simulink model "WristIdentScheme"  (R2025b)
settings: Solver=FixedStepAuto  StartTime=0.0  StopTime=10  FixedStep=1e-3  RelTol=1e-3
model workspace: external: MATLAB File WristAssembly_DataFile.m (data not in the file)
undefined symbols (not defined in the file): smiData, X, Y, Z
libraries: sm_lib x20, nesl_utility x16
settings Model: Creator=Asus  LastModifiedBy=Asus

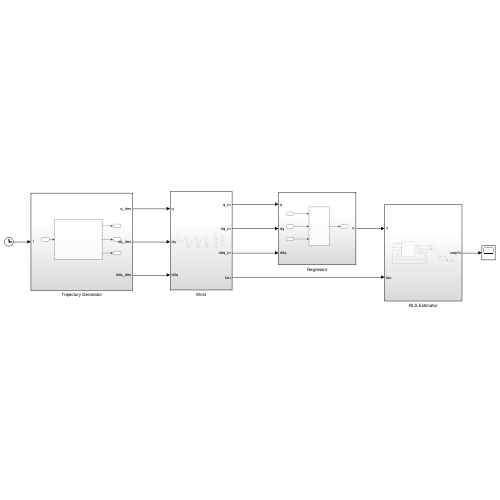
[thumbnail: Simulink's stored preview of the top-level diagram]
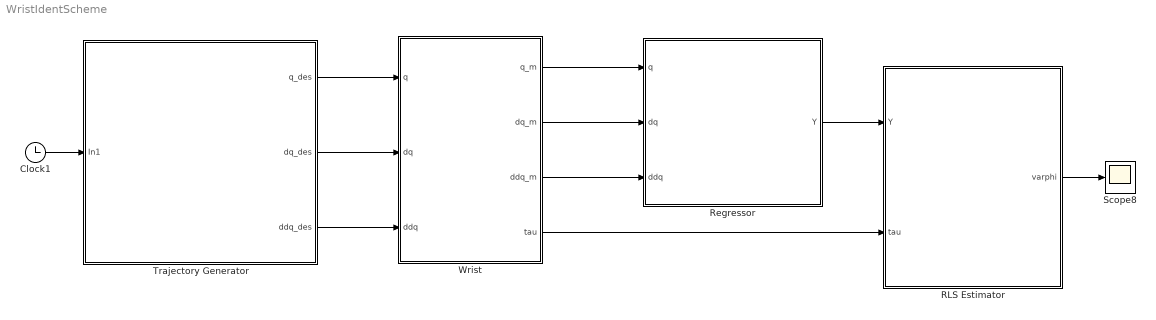
== system WristIdentScheme ==
  Clock1 : Clock
  RLS Estimator : Subsystem
  Regressor : Subsystem
  Scope8 : Scope
      settings: ActiveDisplayYMinimum=-8.9167917961157173  ActiveDisplayYMaximum=6.4052375907209349  DataLoggingVariableName=ScopeData12
  Trajectory Generator : Subsystem
  Wrist : Subsystem
  wires:
  Regressor/1(Y) -> RLS Estimator/1(Y)
  RLS Estimator/1(varphi) -> Scope8/1
  Wrist/1(q_m) -> Regressor/1(q)
  Wrist/2(dq_m) -> Regressor/2(dq)
  Wrist/3(ddq_m) -> Regressor/3(ddq)
  Wrist/4(tau) -> RLS Estimator/2(tau)
  Clock1/1 -> Trajectory Generator/1(In1)
  Trajectory Generator/2(dq_des) -> Wrist/2(dq)
  Trajectory Generator/1(q_des) -> Wrist/1(q)
  Trajectory Generator/3(ddq_des) -> Wrist/3(ddq)

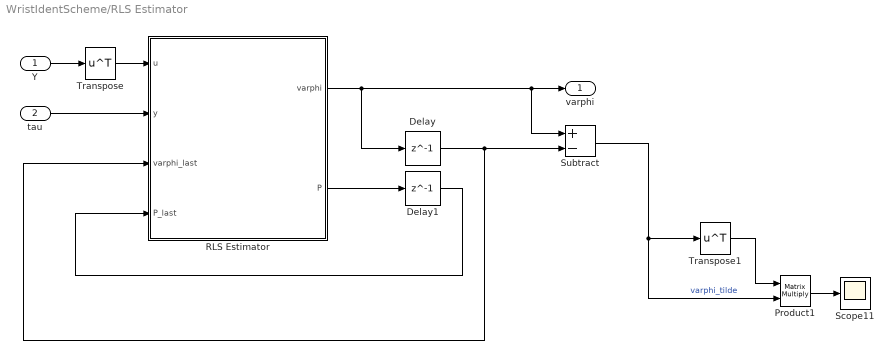
== system WristIdentScheme/RLS Estimator ==
  Y : Inport
  tau : Inport  Port=2
  Delay : Delay  DelayLength=1  InitialCondition=zeros(12, 1)
  Delay1 : Delay  DelayLength=1  InitialCondition=1e+4 * eye(12)
  Product1 : Product  Multiplication=Matrix(*)
  RLS Estimator : MATLAB Function  TreatAsAtomicUnit=on
  Scope11 : Scope
      settings: ActiveDisplayYMinimum=-1.1979056789064427E-9  ActiveDisplayYMaximum=5.9268912686595225E-10  DataLoggingVariableName=ScopeData14
  Subtract : Sum  Inputs=+-
  Transpose : Math  Operator=transpose
  Transpose1 : Math  Operator=transpose
  varphi : Outport
  wires:
  Y/1 -> Transpose/1
  tau/1 -> RLS Estimator/2(y)
  RLS Estimator/1(varphi) -> Subtract/1, varphi/1, Delay/1
  Delay/1 -> RLS Estimator/3(varphi_last), Subtract/2
  RLS Estimator/2(P) -> Delay1/1
  Delay1/1 -> RLS Estimator/4(P_last)
  Transpose/1 -> RLS Estimator/1(u)
  Transpose1/1 -> Product1/1
  Product1/1 -> Scope11/1
  Subtract/1 -> Transpose1/1, Product1/2  "varphi_tilde"

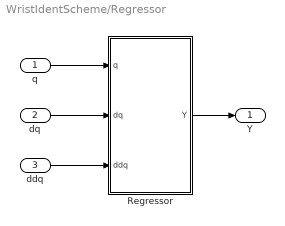
== system WristIdentScheme/Regressor ==
  q : Inport
  dq : Inport  Port=2
  ddq : Inport  Port=3
  Regressor : MATLAB Function  TreatAsAtomicUnit=on
  Y : Outport
  wires:
  q/1 -> Regressor/1(q)
  dq/1 -> Regressor/2(dq)
  ddq/1 -> Regressor/3(ddq)
  Regressor/1(Y) -> Y/1

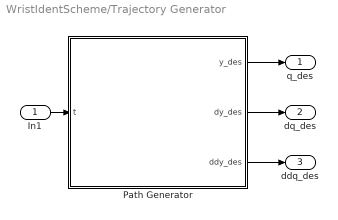
== system WristIdentScheme/Trajectory Generator ==
  In1 : Inport
  Path Generator : MATLAB Function  TreatAsAtomicUnit=on
  q_des : Outport
  dq_des : Outport  Port=2
  ddq_des : Outport  Port=3
  wires:
  In1/1 -> Path Generator/1(t)
  Path Generator/1(y_des) -> q_des/1
  Path Generator/2(dy_des) -> dq_des/1
  Path Generator/3(ddy_des) -> ddq_des/1

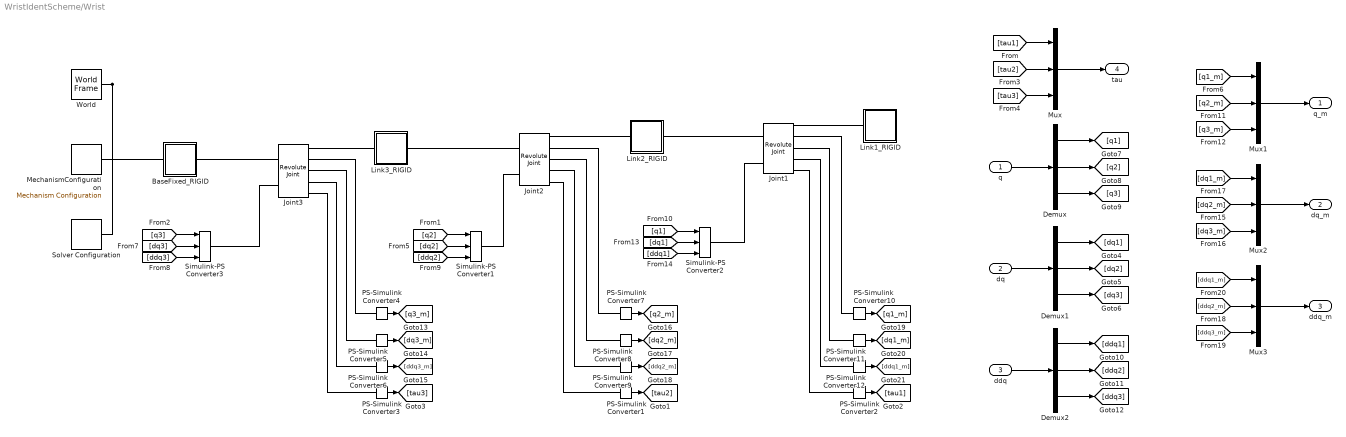
== system WristIdentScheme/Wrist ==
  q : Inport
  dq : Inport  Port=2
  ddq : Inport  Port=3
  BaseFixed_RIGID : Subsystem
  Demux : Demux  Outputs=3
  Demux1 : Demux  Outputs=3
  Demux2 : Demux  Outputs=3
  Joint1 : sm_lib/Joints/Revolute Joint  JointMode=Normal  CompositeWrenchDir=FollowerOnBase  CompositeWrenchFrame=BaseFrame  SenseConstraintForce=off  SenseConstraintTorque=off  SenseTotalForce=off  SenseTotalTorque=off  PositionTargetSpecify=on  PositionTargetPriority=Low  PositionTargetValue=smiData.RevoluteJoint(1).Rz.Pos  PositionTargetValueUnits=deg  VelocityTargetSpecify=off  VelocityTargetPriority=High  VelocityTargetValue=0  VelocityTargetValueUnits=deg/s  EquilibriumPosition=0  EquilibriumPositionUnits=deg  SpringStiffness=0  SpringStiffnessUnits=N*m/deg  DampingCoefficient=0  DampingCoefficientUnits=N*m/(deg/s)  LowerLimitSpecify=off  LowerLimitBound=-90  LowerLimitBoundUnits=deg  LowerLimitStiffness=1e4  LowerLimitStiffnessUnits=N*m/deg  LowerLimitDamping=10  LowerLimitDampingUnits=N*m/(deg/s)  LowerLimitTransitionRegionWidth=0.1  LowerLimitTransitionRegionWidthUnits=deg  UpperLimitSpecify=off  UpperLimitBound=90  UpperLimitBoundUnits=deg  UpperLimitStiffness=1e4  UpperLimitStiffnessUnits=N*m/deg  UpperLimitDamping=10  UpperLimitDampingUnits=N*m/(deg/s)  UpperLimitTransitionRegionWidth=0.1  UpperLimitTransitionRegionWidthUnits=deg  TorqueActuationMode=ComputedTorque  MotionActuationMode=InputMotion  SensePosition=on  SenseVelocity=on  SenseAcceleration=on  SenseTorqueForce=on  SenseLowerLimitTorqueForce=off  SenseUpperLimitTorqueForce=off
  Joint2 : sm_lib/Joints/Revolute Joint  JointMode=Normal  CompositeWrenchDir=FollowerOnBase  CompositeWrenchFrame=BaseFrame  SenseConstraintForce=off  SenseConstraintTorque=off  SenseTotalForce=off  SenseTotalTorque=off  PositionTargetSpecify=on  PositionTargetPriority=Low  PositionTargetValue=smiData.RevoluteJoint(2).Rz.Pos  PositionTargetValueUnits=deg  VelocityTargetSpecify=off  VelocityTargetPriority=High  VelocityTargetValue=0  VelocityTargetValueUnits=deg/s  EquilibriumPosition=0  EquilibriumPositionUnits=deg  SpringStiffness=0  SpringStiffnessUnits=N*m/deg  DampingCoefficient=0  DampingCoefficientUnits=N*m/(deg/s)  LowerLimitSpecify=off  LowerLimitBound=-90  LowerLimitBoundUnits=deg  LowerLimitStiffness=1e4  LowerLimitStiffnessUnits=N*m/deg  LowerLimitDamping=10  LowerLimitDampingUnits=N*m/(deg/s)  LowerLimitTransitionRegionWidth=0.1  LowerLimitTransitionRegionWidthUnits=deg  UpperLimitSpecify=off  UpperLimitBound=90  UpperLimitBoundUnits=deg  UpperLimitStiffness=1e4  UpperLimitStiffnessUnits=N*m/deg  UpperLimitDamping=10  UpperLimitDampingUnits=N*m/(deg/s)  UpperLimitTransitionRegionWidth=0.1  UpperLimitTransitionRegionWidthUnits=deg  TorqueActuationMode=ComputedTorque  MotionActuationMode=InputMotion  SensePosition=on  SenseVelocity=on  SenseAcceleration=on  SenseTorqueForce=on  SenseLowerLimitTorqueForce=off  SenseUpperLimitTorqueForce=off
  Joint3 : sm_lib/Joints/Revolute Joint  JointMode=Normal  CompositeWrenchDir=FollowerOnBase  CompositeWrenchFrame=BaseFrame  SenseConstraintForce=off  SenseConstraintTorque=off  SenseTotalForce=off  SenseTotalTorque=off  PositionTargetSpecify=on  PositionTargetPriority=Low  PositionTargetValue=smiData.RevoluteJoint(3).Rz.Pos  PositionTargetValueUnits=deg  VelocityTargetSpecify=off  VelocityTargetPriority=High  VelocityTargetValue=0  VelocityTargetValueUnits=deg/s  EquilibriumPosition=0  EquilibriumPositionUnits=deg  SpringStiffness=0  SpringStiffnessUnits=N*m/deg  DampingCoefficient=0  DampingCoefficientUnits=N*m/(deg/s)  LowerLimitSpecify=off  LowerLimitBound=-90  LowerLimitBoundUnits=deg  LowerLimitStiffness=1e4  LowerLimitStiffnessUnits=N*m/deg  LowerLimitDamping=10  LowerLimitDampingUnits=N*m/(deg/s)  LowerLimitTransitionRegionWidth=0.1  LowerLimitTransitionRegionWidthUnits=deg  UpperLimitSpecify=off  UpperLimitBound=90  UpperLimitBoundUnits=deg  UpperLimitStiffness=1e4  UpperLimitStiffnessUnits=N*m/deg  UpperLimitDamping=10  UpperLimitDampingUnits=N*m/(deg/s)  UpperLimitTransitionRegionWidth=0.1  UpperLimitTransitionRegionWidthUnits=deg  TorqueActuationMode=ComputedTorque  MotionActuationMode=InputMotion  SensePosition=on  SenseVelocity=on  SenseAcceleration=on  SenseTorqueForce=on  SenseLowerLimitTorqueForce=off  SenseUpperLimitTorqueForce=off
  Link1_RIGID : Subsystem
  Link2_RIGID : Subsystem
  Link3_RIGID : Subsystem
  MechanismConfiguration : sm_lib/Utilities/Mechanism Configuration  UniformGravity=Constant  GravityVector=[0 0 -9.80665] * 1  GravityVectorUnits=m/s^2  LinearizationDelta=0.001  JointModeTransitionNonlinearIterations=2
  Mux{,1..3} (4 alike) : Mux  Inputs=3
  PS-Simulink Converter1 : nesl_utility/PS-Simulink Converter  PhysicalDomain=network_engine_domain  SubClassName=ps_output  LeftPortType=input  RightPortType=output  PseudoPeriodic=off  Frequencies=[]  VectorFormat=inherit  Unit=N*m  AffineConversion=off
  PS-Simulink Converter10 : nesl_utility/PS-Simulink Converter  PhysicalDomain=network_engine_domain  SubClassName=ps_output  LeftPortType=input  RightPortType=output  PseudoPeriodic=off  Frequencies=[]  VectorFormat=inherit  Unit=rad  AffineConversion=off
  PS-Simulink Converter11 : nesl_utility/PS-Simulink Converter  PhysicalDomain=network_engine_domain  SubClassName=ps_output  LeftPortType=input  RightPortType=output  PseudoPeriodic=off  Frequencies=[]  VectorFormat=inherit  Unit=rad/s  AffineConversion=off
  PS-Simulink Converter12 : nesl_utility/PS-Simulink Converter  PhysicalDomain=network_engine_domain  SubClassName=ps_output  LeftPortType=input  RightPortType=output  PseudoPeriodic=off  Frequencies=[]  VectorFormat=inherit  Unit=rad/s^2  AffineConversion=off
  PS-Simulink Converter2 : nesl_utility/PS-Simulink Converter  PhysicalDomain=network_engine_domain  SubClassName=ps_output  LeftPortType=input  RightPortType=output  PseudoPeriodic=off  Frequencies=[]  VectorFormat=inherit  Unit=N*m  AffineConversion=off
  PS-Simulink Converter3 : nesl_utility/PS-Simulink Converter  PhysicalDomain=network_engine_domain  SubClassName=ps_output  LeftPortType=input  RightPortType=output  PseudoPeriodic=off  Frequencies=[]  VectorFormat=inherit  Unit=N*m  AffineConversion=off
  PS-Simulink Converter4 : nesl_utility/PS-Simulink Converter  PhysicalDomain=network_engine_domain  SubClassName=ps_output  LeftPortType=input  RightPortType=output  PseudoPeriodic=off  Frequencies=[]  VectorFormat=inherit  Unit=rad  AffineConversion=off
  PS-Simulink Converter5 : nesl_utility/PS-Simulink Converter  PhysicalDomain=network_engine_domain  SubClassName=ps_output  LeftPortType=input  RightPortType=output  PseudoPeriodic=off  Frequencies=[]  VectorFormat=inherit  Unit=rad/s  AffineConversion=off
  PS-Simulink Converter6 : nesl_utility/PS-Simulink Converter  PhysicalDomain=network_engine_domain  SubClassName=ps_output  LeftPortType=input  RightPortType=output  PseudoPeriodic=off  Frequencies=[]  VectorFormat=inherit  Unit=rad/s^2  AffineConversion=off
  PS-Simulink Converter7 : nesl_utility/PS-Simulink Converter  PhysicalDomain=network_engine_domain  SubClassName=ps_output  LeftPortType=input  RightPortType=output  PseudoPeriodic=off  Frequencies=[]  VectorFormat=inherit  Unit=rad  AffineConversion=off
  PS-Simulink Converter8 : nesl_utility/PS-Simulink Converter  PhysicalDomain=network_engine_domain  SubClassName=ps_output  LeftPortType=input  RightPortType=output  PseudoPeriodic=off  Frequencies=[]  VectorFormat=inherit  Unit=rad/s  AffineConversion=off
  PS-Simulink Converter9 : nesl_utility/PS-Simulink Converter  PhysicalDomain=network_engine_domain  SubClassName=ps_output  LeftPortType=input  RightPortType=output  PseudoPeriodic=off  Frequencies=[]  VectorFormat=inherit  Unit=rad/s^2  AffineConversion=off
  Simulink-PS Converter1 : nesl_utility/Simulink-PS Converter  PhysicalDomain=network_engine_domain  SubClassName=ps_input  LeftPortType=input  RightPortType=output  PseudoPeriodic=off  Frequencies=[]  NoiseDistribution=none  NoiseParameters=[]  Unit=rad  AffineConversion=off  FilteringAndDerivatives=provide  SimscapeFilterOrder=1  InputFilterTimeConstant=0.001  UdotUserProvided=2
  Simulink-PS Converter2 : nesl_utility/Simulink-PS Converter  PhysicalDomain=network_engine_domain  SubClassName=ps_input  LeftPortType=input  RightPortType=output  PseudoPeriodic=off  Frequencies=[]  NoiseDistribution=none  NoiseParameters=[]  Unit=rad  AffineConversion=off  FilteringAndDerivatives=provide  SimscapeFilterOrder=1  InputFilterTimeConstant=0.001  UdotUserProvided=2
  Simulink-PS Converter3 : nesl_utility/Simulink-PS Converter  PhysicalDomain=network_engine_domain  SubClassName=ps_input  LeftPortType=input  RightPortType=output  PseudoPeriodic=off  Frequencies=[]  NoiseDistribution=none  NoiseParameters=[]  Unit=rad  AffineConversion=off  FilteringAndDerivatives=provide  SimscapeFilterOrder=1  InputFilterTimeConstant=0.001  UdotUserProvided=2
  Solver Configuration : nesl_utility/Solver Configuration  PhysicalDomain=network_engine_domain  SubClassName=solver  LeftPortType=input  RightPortType=generic  Tones=[]  Harmonics=[]  SimulateNoise=off  Profile=off  UseLocalSampling=off  EnableSwitchedLinearOptims=on  FrequencyDomain=off  UseCCode=off  RelTol=0.001  AbsTol=0.001  MinStep=1e-09  ToWorkspace=off  RevertToSquareIcSolve=off  NumHomotopyIterations=100  PhasorMode=off  PhasorModeNumHarmonics=1  ConsistencySolver=NEWTON_XTOL_AFTER_FTOL  IndexReductionMethod=DerivativeReplacement  DoDC=off  ResidualTolerance=1e-09  ConsistencyTolSource=GLOBAL  ConsistencyAbsTol=0.001  ConsistencyRelTol=0.001  ConsistencyTolFactor=0.001  UseLocalSolver=off  LocalSolverChoice=NE_BACKWARD_EULER_ADVANCER  ResolveIndetEquations=on  FunctionEvalNumThread=1  LocalSolverSampleTime=0.001  DoFixedCost=off  MaxNonlinIter=3  MaxModeIter=2  ComputeImpulses=off  ImpulseIterations=2  LinearAlgebra=auto  LinearAlgebraNumThread=0  EquationFormulation=NE_TIME_EF  DelaysMemoryBudget=1024  AutomaticFiltering=on  FilteringTimeConstant=0.001  PartitionStorageMethod=AS_NEEDED  PartitionMemoryBudget=1024  PartitionMethod=ROBUST  MultibodyUseLocalSolver=off  MultibodyLocalSolverChoice=ODE1  MultibodyLocalSolverSampleTime=0.001
  World : sm_lib/Frames and Transforms/World Frame
  q_m : Outport
  dq_m : Outport  Port=2
  ddq_m : Outport  Port=3
  tau : Outport  Port=4
  wires:
  PS-Simulink Converter3/1 -> [tau3]
  PS-Simulink Converter1/1 -> [tau2]
  PS-Simulink Converter2/1 -> [tau1]
  [tau3] -> Mux/3
  Mux/1 -> tau/1
  Demux2/3 -> [ddq3]
  Demux1/2 -> [dq2]
  Demux/3 -> [q3]
  q/1 -> Demux/1
  ddq/1 -> Demux2/1
  Demux/2 -> [q2]
  Demux1/1 -> [dq1]
  [tau2] -> Mux/2
  Demux/1 -> [q1]
  Demux2/1 -> [ddq1]
  Demux2/2 -> [ddq2]
  Demux1/3 -> [dq3]
  [tau1] -> Mux/1
  dq/1 -> Demux1/1
  PS-Simulink Converter4/1 -> [q3_m]
  PS-Simulink Converter5/1 -> [dq3_m]
  PS-Simulink Converter6/1 -> [ddq3_m]
  PS-Simulink Converter9/1 -> [ddq2_m]
  PS-Simulink Converter7/1 -> [q2_m]
  PS-Simulink Converter8/1 -> [dq2_m]
  PS-Simulink Converter12/1 -> [ddq1_m]
  PS-Simulink Converter10/1 -> [q1_m]
  PS-Simulink Converter11/1 -> [dq1_m]
  Mux1/1 -> q_m/1
  [q1_m] -> Mux1/1
  [q2_m] -> Mux1/2
  [q3_m] -> Mux1/3
  Mux2/1 -> dq_m/1
  [dq1_m] -> Mux2/1
  [dq3_m] -> Mux2/3
  [dq2_m] -> Mux2/2
  [ddq1_m] -> Mux3/1
  Mux3/1 -> ddq_m/1
  [ddq3_m] -> Mux3/3
  [ddq2_m] -> Mux3/2
  [q3] -> Simulink-PS Converter3/1
  [dq3] -> Simulink-PS Converter3/2
  [ddq3] -> Simulink-PS Converter3/3
  [dq2] -> Simulink-PS Converter1/2
  [q2] -> Simulink-PS Converter1/1
  [ddq2] -> Simulink-PS Converter1/3
  [q1] -> Simulink-PS Converter2/1
  [ddq1] -> Simulink-PS Converter2/3
  [dq1] -> Simulink-PS Converter2/2
  connections:
  Link3_RIGID/RConn1 -- Joint2/LConn1
  World/RConn1 -- BaseFixed_RIGID/LConn1 -- Solver Configuration/RConn1 -- MechanismConfiguration/RConn1
  BaseFixed_RIGID/RConn1 -- Joint3/LConn1
  Link2_RIGID/RConn1 -- Joint1/LConn1
  Link3_RIGID/LConn1 -- Joint3/RConn1
  Link2_RIGID/LConn1 -- Joint2/RConn1
  Link1_RIGID/LConn1 -- Joint1/RConn1
  Simulink-PS Converter3/RConn1 -- Joint3/LConn2
  PS-Simulink Converter3/LConn1 -- Joint3/RConn5
  Simulink-PS Converter1/RConn1 -- Joint2/LConn2
  PS-Simulink Converter1/LConn1 -- Joint2/RConn5
  Simulink-PS Converter2/RConn1 -- Joint1/LConn2
  PS-Simulink Converter2/LConn1 -- Joint1/RConn5
  PS-Simulink Converter4/LConn1 -- Joint3/RConn2
  PS-Simulink Converter5/LConn1 -- Joint3/RConn3
  PS-Simulink Converter6/LConn1 -- Joint3/RConn4
  PS-Simulink Converter7/LConn1 -- Joint2/RConn2
  PS-Simulink Converter8/LConn1 -- Joint2/RConn3
  PS-Simulink Converter9/LConn1 -- Joint2/RConn4
  PS-Simulink Converter10/LConn1 -- Joint1/RConn2
  PS-Simulink Converter11/LConn1 -- Joint1/RConn3
  PS-Simulink Converter12/LConn1 -- Joint1/RConn4

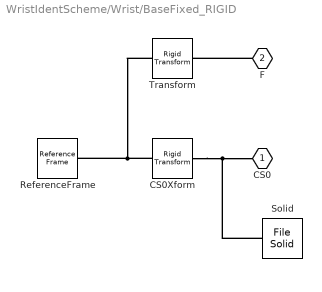
== system WristIdentScheme/Wrist/BaseFixed_RIGID ==
  CS0Xform : sm_lib/Frames and Transforms/Rigid Transform  RotationMethod=ArbitraryAxis  FollAlignAxisA=+X  BaseAlignAxisA=+Y  FollAlignAxisB=+Y  BaseAlignAxisB=+Z  RotationStandardAxis=+Z  RotationAngle=smiData.RigidTransform(3).angle  RotationAngleUnits=rad  RotationArbitraryAxis=smiData.RigidTransform(3).axis  RotationSequenceAxes=FollowerAxes  RotationSequence=XYX  RotationSequenceAngles=[0 0 0]  RotationSequenceAnglesUnits=deg  RotationMatrix=[1 0 0;0 1 0;0 0 1]  Quaternion=[1 0 0 0]  TranslationMethod=Cartesian  TranslationCartesianOffset=smiData.RigidTransform(3).translation  TranslationCartesianOffsetUnits=mm  TranslationStandardAxis=+Z  TranslationStandardOffset=0  TranslationStandardOffsetUnits=m  TranslationROffset=0  TranslationROffsetUnits=m  TranslationThetaOffset=0  TranslationThetaOffsetUnits=deg  TranslationZOffset=0  TranslationZOffsetUnits=m
  ReferenceFrame : sm_lib/Frames and Transforms/Reference Frame
  Solid : sm_lib/Body Elements/File Solid  ExtGeomFileName=BaseFixed.STEP  UnitType=FromFile  ExtGeomFileUnits=m  StepReaderType=HEX  ExportConvexHullGeometry=off  InertiaType=Custom  BasedOnType=DensityFromFile  Density=1000  DensityUnits=kg/m^3  Mass=smiData.BaseFixed.mass  MassUnits=kg  CenterOfMass=smiData.BaseFixed.CoM  CenterOfMassUnits=mm  MomentsOfInertia=smiData.BaseFixed.MoI  MomentsOfInertiaUnits=kg*mm^2  ProductsOfInertia=smiData.BaseFixed.PoI  ProductsOfInertiaUnits=kg*mm^2  GraphicType=FromGeometry  MarkerShape=Sphere  MarkerSize=10  GraphicVisPropType=SimpleVisualProperties  GraphicDiffuseColor=smiData.Solid(14).color  GraphicOpacity=smiData.Solid(14).opacity  GraphicSpecularColor=[0.5 0.5 0.5 1.0]  GraphicAmbientColor=[0.15 0.15 0.15 1.0]  GraphicEmissiveColor=[0.0 0.0 0.0 1.0]  GraphicShininess=75  DoExposeReferenceFrame=on  SerializedFrames=<Frames/>
  Transform : sm_lib/Frames and Transforms/Rigid Transform  RotationMethod=ArbitraryAxis  FollAlignAxisA=+X  BaseAlignAxisA=+Y  FollAlignAxisB=+Y  BaseAlignAxisB=+Z  RotationStandardAxis=+Z  RotationAngle=smiData.RigidTransform(10).angle  RotationAngleUnits=rad  RotationArbitraryAxis=smiData.RigidTransform(10).axis  RotationSequenceAxes=FollowerAxes  RotationSequence=XYX  RotationSequenceAngles=[0 0 0]  RotationSequenceAnglesUnits=deg  RotationMatrix=[1 0 0;0 1 0;0 0 1]  Quaternion=[1 0 0 0]  TranslationMethod=Cartesian  TranslationCartesianOffset=smiData.RigidTransform(10).translation  TranslationCartesianOffsetUnits=mm  TranslationStandardAxis=+Z  TranslationStandardOffset=0  TranslationStandardOffsetUnits=m  TranslationROffset=0  TranslationROffsetUnits=m  TranslationThetaOffset=0  TranslationThetaOffsetUnits=deg  TranslationZOffset=0  TranslationZOffsetUnits=m
  CS0 : PMIOPort  Side=Left
  F : PMIOPort  Port=2  Side=Right
  connections:
  CS0Xform/RConn1 -- Solid/RConn1 -- CS0/RConn1
  CS0Xform/LConn1 -- Transform/LConn1 -- ReferenceFrame/RConn1
  F/RConn1 -- Transform/RConn1

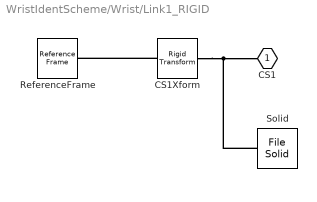
== system WristIdentScheme/Wrist/Link1_RIGID ==
  CS1Xform : sm_lib/Frames and Transforms/Rigid Transform  RotationMethod=ArbitraryAxis  FollAlignAxisA=+X  BaseAlignAxisA=+Y  FollAlignAxisB=+Y  BaseAlignAxisB=+Z  RotationStandardAxis=+Z  RotationAngle=smiData.RigidTransform(2).angle  RotationAngleUnits=rad  RotationArbitraryAxis=smiData.RigidTransform(2).axis  RotationSequenceAxes=FollowerAxes  RotationSequence=XYX  RotationSequenceAngles=[0 0 0]  RotationSequenceAnglesUnits=deg  RotationMatrix=[1 0 0;0 1 0;0 0 1]  Quaternion=[1 0 0 0]  TranslationMethod=Cartesian  TranslationCartesianOffset=smiData.RigidTransform(2).translation  TranslationCartesianOffsetUnits=mm  TranslationStandardAxis=+Z  TranslationStandardOffset=0  TranslationStandardOffsetUnits=m  TranslationROffset=0  TranslationROffsetUnits=m  TranslationThetaOffset=0  TranslationThetaOffsetUnits=deg  TranslationZOffset=0  TranslationZOffsetUnits=m
  ReferenceFrame : sm_lib/Frames and Transforms/Reference Frame
  Solid : sm_lib/Body Elements/File Solid  ExtGeomFileName=Link1.STEP  UnitType=FromFile  ExtGeomFileUnits=m  StepReaderType=HEX  ExportConvexHullGeometry=off  InertiaType=Custom  BasedOnType=DensityFromFile  Density=1000  DensityUnits=kg/m^3  Mass=smiData.Link1.mass  MassUnits=kg  CenterOfMass=smiData.Link1.CoM  CenterOfMassUnits=mm  MomentsOfInertia=smiData.Link1.MoI  MomentsOfInertiaUnits=kg*mm^2  ProductsOfInertia=smiData.Link1.PoI  ProductsOfInertiaUnits=kg*mm^2  GraphicType=FromGeometry  MarkerShape=Sphere  MarkerSize=10  GraphicVisPropType=SimpleVisualProperties  GraphicDiffuseColor=smiData.Solid(14).color  GraphicOpacity=smiData.Solid(14).opacity  GraphicSpecularColor=[0.5 0.5 0.5 1.0]  GraphicAmbientColor=[0.15 0.15 0.15 1.0]  GraphicEmissiveColor=[0.0 0.0 0.0 1.0]  GraphicShininess=75  DoExposeReferenceFrame=on  SerializedFrames=<Frames/>
  CS1 : PMIOPort  Side=Left
  connections:
  CS1Xform/LConn1 -- ReferenceFrame/RConn1
  CS1Xform/RConn1 -- Solid/RConn1 -- CS1/RConn1

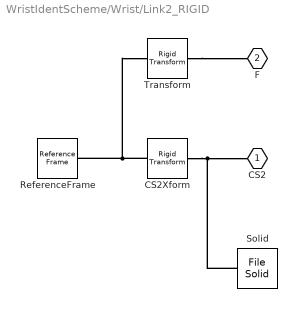
== system WristIdentScheme/Wrist/Link2_RIGID ==
  CS2Xform : sm_lib/Frames and Transforms/Rigid Transform  RotationMethod=ArbitraryAxis  FollAlignAxisA=+X  BaseAlignAxisA=+Y  FollAlignAxisB=+Y  BaseAlignAxisB=+Z  RotationStandardAxis=+Z  RotationAngle=smiData.RigidTransform(4).angle  RotationAngleUnits=rad  RotationArbitraryAxis=smiData.RigidTransform(4).axis  RotationSequenceAxes=FollowerAxes  RotationSequence=XYX  RotationSequenceAngles=[0 0 0]  RotationSequenceAnglesUnits=deg  RotationMatrix=[1 0 0;0 1 0;0 0 1]  Quaternion=[1 0 0 0]  TranslationMethod=Cartesian  TranslationCartesianOffset=smiData.RigidTransform(4).translation  TranslationCartesianOffsetUnits=mm  TranslationStandardAxis=+Z  TranslationStandardOffset=0  TranslationStandardOffsetUnits=m  TranslationROffset=0  TranslationROffsetUnits=m  TranslationThetaOffset=0  TranslationThetaOffsetUnits=deg  TranslationZOffset=0  TranslationZOffsetUnits=m
  ReferenceFrame : sm_lib/Frames and Transforms/Reference Frame
  Solid : sm_lib/Body Elements/File Solid  ExtGeomFileName=Link2.STEP  UnitType=FromFile  ExtGeomFileUnits=m  StepReaderType=HEX  ExportConvexHullGeometry=off  InertiaType=Custom  BasedOnType=DensityFromFile  Density=1000  DensityUnits=kg/m^3  Mass=smiData.Link2.mass  MassUnits=kg  CenterOfMass=smiData.Link2.CoM  CenterOfMassUnits=mm  MomentsOfInertia=smiData.Link2.MoI  MomentsOfInertiaUnits=kg*mm^2  ProductsOfInertia=smiData.Link2.PoI  ProductsOfInertiaUnits=kg*mm^2  GraphicType=FromGeometry  MarkerShape=Sphere  MarkerSize=10  GraphicVisPropType=SimpleVisualProperties  GraphicDiffuseColor=smiData.Solid(14).color  GraphicOpacity=smiData.Solid(14).opacity  GraphicSpecularColor=[0.5 0.5 0.5 1.0]  GraphicAmbientColor=[0.15 0.15 0.15 1.0]  GraphicEmissiveColor=[0.0 0.0 0.0 1.0]  GraphicShininess=75  DoExposeReferenceFrame=on  SerializedFrames=<Frames/>
  Transform : sm_lib/Frames and Transforms/Rigid Transform  RotationMethod=ArbitraryAxis  FollAlignAxisA=+X  BaseAlignAxisA=+Y  FollAlignAxisB=+Y  BaseAlignAxisB=+Z  RotationStandardAxis=+Z  RotationAngle=smiData.RigidTransform(6).angle  RotationAngleUnits=rad  RotationArbitraryAxis=smiData.RigidTransform(6).axis  RotationSequenceAxes=FollowerAxes  RotationSequence=XYX  RotationSequenceAngles=[0 0 0]  RotationSequenceAnglesUnits=deg  RotationMatrix=[1 0 0;0 1 0;0 0 1]  Quaternion=[1 0 0 0]  TranslationMethod=Cartesian  TranslationCartesianOffset=smiData.RigidTransform(6).translation  TranslationCartesianOffsetUnits=mm  TranslationStandardAxis=+Z  TranslationStandardOffset=0  TranslationStandardOffsetUnits=m  TranslationROffset=0  TranslationROffsetUnits=m  TranslationThetaOffset=0  TranslationThetaOffsetUnits=deg  TranslationZOffset=0  TranslationZOffsetUnits=m
  CS2 : PMIOPort  Side=Left
  F : PMIOPort  Port=2  Side=Right
  connections:
  ReferenceFrame/RConn1 -- CS2Xform/LConn1 -- Transform/LConn1
  CS2Xform/RConn1 -- Solid/RConn1 -- CS2/RConn1
  Transform/RConn1 -- F/RConn1

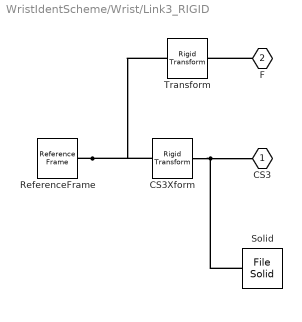
== system WristIdentScheme/Wrist/Link3_RIGID ==
  CS3Xform : sm_lib/Frames and Transforms/Rigid Transform  RotationMethod=ArbitraryAxis  FollAlignAxisA=+X  BaseAlignAxisA=+Y  FollAlignAxisB=+Y  BaseAlignAxisB=+Z  RotationStandardAxis=+Z  RotationAngle=smiData.RigidTransform(1).angle  RotationAngleUnits=rad  RotationArbitraryAxis=smiData.RigidTransform(1).axis  RotationSequenceAxes=FollowerAxes  RotationSequence=XYX  RotationSequenceAngles=[0 0 0]  RotationSequenceAnglesUnits=deg  RotationMatrix=[1 0 0;0 1 0;0 0 1]  Quaternion=[1 0 0 0]  TranslationMethod=Cartesian  TranslationCartesianOffset=smiData.RigidTransform(1).translation  TranslationCartesianOffsetUnits=mm  TranslationStandardAxis=+Z  TranslationStandardOffset=0  TranslationStandardOffsetUnits=m  TranslationROffset=0  TranslationROffsetUnits=m  TranslationThetaOffset=0  TranslationThetaOffsetUnits=deg  TranslationZOffset=0  TranslationZOffsetUnits=m
  ReferenceFrame : sm_lib/Frames and Transforms/Reference Frame
  Solid : sm_lib/Body Elements/File Solid  ExtGeomFileName=Link3.STEP  UnitType=FromFile  ExtGeomFileUnits=m  StepReaderType=HEX  ExportConvexHullGeometry=off  InertiaType=Custom  BasedOnType=DensityFromFile  Density=1000  DensityUnits=kg/m^3  Mass=smiData.Link3.mass  MassUnits=kg  CenterOfMass=smiData.Link3.CoM  CenterOfMassUnits=mm  MomentsOfInertia=smiData.Link3.MoI  MomentsOfInertiaUnits=kg*mm^2  ProductsOfInertia=smiData.Link3.PoI  ProductsOfInertiaUnits=kg*mm^2  GraphicType=FromGeometry  MarkerShape=Sphere  MarkerSize=10  GraphicVisPropType=SimpleVisualProperties  GraphicDiffuseColor=smiData.Solid(14).color  GraphicOpacity=smiData.Solid(14).opacity  GraphicSpecularColor=[0.5 0.5 0.5 1.0]  GraphicAmbientColor=[0.15 0.15 0.15 1.0]  GraphicEmissiveColor=[0.0 0.0 0.0 1.0]  GraphicShininess=75  DoExposeReferenceFrame=on  SerializedFrames=<Frames/>
  Transform : sm_lib/Frames and Transforms/Rigid Transform  RotationMethod=ArbitraryAxis  FollAlignAxisA=+X  BaseAlignAxisA=+Y  FollAlignAxisB=+Y  BaseAlignAxisB=+Z  RotationStandardAxis=+Z  RotationAngle=smiData.RigidTransform(7).angle  RotationAngleUnits=rad  RotationArbitraryAxis=smiData.RigidTransform(7).axis  RotationSequenceAxes=FollowerAxes  RotationSequence=XYX  RotationSequenceAngles=[0 0 0]  RotationSequenceAnglesUnits=deg  RotationMatrix=[1 0 0;0 1 0;0 0 1]  Quaternion=[1 0 0 0]  TranslationMethod=Cartesian  TranslationCartesianOffset=smiData.RigidTransform(7).translation  TranslationCartesianOffsetUnits=mm  TranslationStandardAxis=+Z  TranslationStandardOffset=0  TranslationStandardOffsetUnits=m  TranslationROffset=0  TranslationROffsetUnits=m  TranslationThetaOffset=0  TranslationThetaOffsetUnits=deg  TranslationZOffset=0  TranslationZOffsetUnits=m
  CS3 : PMIOPort  Side=Left
  F : PMIOPort  Port=2  Side=Right
  connections:
  CS3Xform/RConn1 -- Solid/RConn1 -- CS3/RConn1
  ReferenceFrame/RConn1 -- Transform/LConn1 -- CS3Xform/LConn1
  F/RConn1 -- Transform/RConn1

== matlab function WristIdentScheme/Trajectory Generator/Path Generator ==
  data: t input; y_des output; dy_des output; ddy_des output
function [y_des, dy_des, ddy_des] = PathGen(t)


    phi = [4.9930    4.0342    5.9746
    3.6279    2.6330    2.7895
    2.7648    2.4552    0.3771
    1.6186    5.1280    5.4460
    4.7246    1.9945    3.9659
    1.4368    5.1179    2.2310
    0.4033    4.9579    6.2644
    4.8213    5.3549    1.4085
    4.2173    3.1770    4.0995
    4.4938    3.9940    3.8013]';


    w = [3.8823    3.7097    3.9187
    7.2207    7.1975    7.1216
    2.1346    2.2948    2.2197
    3.0818    2.9190    2.9048
    0.6798    0.4240    0.6674
    1.3216    1.2640    1.3458
    5.5778    5.7011    5.3844
    7.9908    7.9062    8.0109
    4.7432    4.6881    4.7056
    6.1853    6.3359    6.3373]';

    A = [1.5418    1.6486    1.6074
    1.5454    1.2746    1.4009
    1.9884    1.9165    1.9476
    2.3471    2.3948    2.3386
    0.6298    0.7054    0.7547
    1.1214    1.1076    1.1863
    0.1257    0.0585    0.1436
    2.4786    2.8080    2.6586
    0.3248    0.6134    0.3718
    3.0841    2.9406    2.9134]';

    maxGain = 2 * [1.5; 0.8; 0.8];
    % maxGain = 1;

    y_des   = zeros(3, 1);
    dy_des  = zeros(3, 1);
    ddy_des = zeros(3, 1);

    for i = 1:10
        y_des   =   y_des + A(:, i)            .*            sin(w(:, i)*t + phi(:, i));
        dy_des  =  dy_des + A(:, i) .* w(:, i) .*            cos(w(:, i)*t + phi(:, i));
        ddy_des = ddy_des - A(:, i) .* w(:, i) .* w(:, i) .* sin(w(:, i)*t + phi(:, i));
    end

    gain = sum(A, 2);

    y_des   =   y_des ./ gain .* maxGain;
    dy_des  =  dy_des ./ gain .* maxGain;
    ddy_des = ddy_des ./ gain .* maxGain;
    
end

% amp  = abs(repmat(linspace(0.1, 3, 10)', 1, 3) + 0.1 * randn(10, 3));
% amp = amp(randperm(10), :)
% 
% freq = abs(repmat(linspace(0.5, 8, 10)', 1, 3) + 0.1 * randn(10, 3));
% freq = freq(randperm(10), :)
% 
% phi = 2 * pi * rand(10, 3)

== matlab function WristIdentScheme/RLS Estimator/RLS Estimator ==
  data: u input; varphi output; y input; varphi_last input; P_last input; P output
function [varphi, P] = fcn(u, y, varphi_last, P_last)

    % estimator gain
    k = (P_last * u) * (eye(3) + u' * P_last * u)^(-1);

    % update estimation params
    varphi = varphi_last + k * (y - u' * varphi_last);

    % update Cov matrix
    P = (eye(12) - k * u') * P_last;
    P = (P + P') / 2;

end

== matlab function WristIdentScheme/Regressor/Regressor ==
  data: q input; Y output; dq input; ddq input
function Y = fcn(q, dq, ddq)

    g = 9.80665;
    
    q1 = q(1); q2 = q(2); q3 = q(3);
    dq1 = dq(1); dq2 = dq(2); dq3 = dq(3);
    ddq1 = ddq(1); ddq2 = ddq(2); ddq3 = ddq(3);
    
    Y = [ddq1*cos(q2)^2*cos(q3)^2 - dq2*((dq3*cos(q2)*(2*cos(q3)^2 - 1))/2 - dq2*cos(q3)*sin(q2)*sin(q3) + dq1*cos(q2)*cos(q3)^2*sin(q2)) - (dq3*cos(q2)*(2*dq2*cos(q3)^2 - dq2 + 2*dq1*cos(q2)*cos(q3)*sin(q3)))/2 - dq1*(dq3*sin(q3)*cos(q2)^2*cos(q3) + dq2*sin(q2)*cos(q2)*cos(q3)^2) - ddq2*cos(q2)*cos(q3)*sin(q3), ddq1*cos(q2)^2 - 2*dq1*dq2*cos(q2)*sin(q2), (ddq2*cos(q3)*sin(q2))/2 - dq2*(dq1*(sin(q3)/2 - cos(q2)^2*sin(q3)) - (dq2*cos(q2)*cos(q3))/2) - (dq3*cos(q2)*(dq3*cos(q3) - dq1*cos(q3)*sin(q2)))/2 - dq1*(dq2*(sin(q3)/2 - cos(q2)^2*sin(q3)) - (dq3*cos(q2)*cos(q3)*sin(q2))/2) - (ddq3*cos(q2)*sin(q3))/2 + ddq1*cos(q2)*sin(q2)*sin(q3), ddq1*cos(q2)*sin(q2) + 2*dq1*dq2*(cos(q2)^2 - 1/2), ddq1, - sin(q2)*dq2^2 + ddq2*cos(q2), cos(q2)*dq2^2 + ddq2*sin(q2),        ddq3*sin(q2) + dq2*dq3*cos(q2),    0,         0,                  0,         0
        dq3*((dq1*cos(q2))/2 + dq2*cos(q3)*sin(q3) - dq1*cos(q2)*cos(q3)^2) + dq1*(dq3*(cos(q2)/2 - cos(q2)*cos(q3)^2) + dq1*cos(q2)*cos(q3)^2*sin(q2)) - ddq2*cos(q3)^2 + (dq2*dq3*sin(2*q3))/2 - ddq1*cos(q2)*cos(q3)*sin(q3),                      dq1^2*cos(q2)*sin(q2),                                                                                                                          dq3*((dq3*sin(q3))/2 - (dq1*sin(q2)*sin(q3))/2) + dq1*(dq1*(sin(q3)/2 - cos(q2)^2*sin(q3)) - (dq3*sin(q2)*sin(q3))/2) - (ddq3*cos(q3))/2 + (ddq1*cos(q3)*sin(q2))/2,                           -dq1^2*(cos(q2)^2 - 1/2),    0,                   ddq1*cos(q2),                 ddq1*sin(q2),                      -dq1*dq3*cos(q2), ddq2, g*cos(q2),  g*sin(q2)*sin(q3), g*sin(q2)
        dq2*(dq1*((cos(q2)*cos(q3)^2)/2 - (cos(q2)*sin(q3)^2)/2) - dq2*cos(q3)*sin(q3)) + dq1*(dq2*((cos(q2)*cos(q3)^2)/2 - (cos(q2)*sin(q3)^2)/2) + dq1*cos(q2)^2*cos(q3)*sin(q3)),                                          0,                                                                                                                                                  dq1*((dq2*sin(q2)*sin(q3))/2 - (dq1*cos(q2)*cos(q3)*sin(q2))/2) - (ddq2*cos(q3))/2 - (ddq1*cos(q2)*sin(q3))/2 + (dq1*dq2*sin(q2)*sin(q3))/2,                                                  0,    0,                              0,                            0, ddq1*sin(q2) - ddq3 + dq1*dq2*cos(q2),    0,         0, -g*cos(q2)*cos(q3),         0];


end
